simulink model "Model_OLD"  (R2024b)
settings: Solver=VariableStepAuto  StartTime=0.0  StopTime=20  MaxStep=0.001  RelTol=1e-4
values from neighbouring files (symbols this model uses):
  A = 1.1    [RT14e_Parameters.m]    (also in RT15e_Parameters.m = 1.088; RT15evo_Parameters.m = 1.088; SIM_setup.m = 1.12)
  Aero_balance = 55    [RT14e_Parameters.m]    (also in RT15e_Parameters.m; RT15evo_Parameters.m; SIM_setup.m = 0.55)
  air_density = 1.29    [SIM_setup.m]
  Br_coef_of_friction_F = 0.33    [RT14e_Parameters.m]    (also in RT15e_Parameters.m; RT15evo_Parameters.m; SIM_setup.m = 0.25)
  Br_coef_of_friction_R = 0.33    [RT14e_Parameters.m]    (also in RT15e_Parameters.m; RT15evo_Parameters.m; SIM_setup.m = 0.25)
  Br_pistons_area_F = 3617.26/1e6    (= 0.00361726)    [RT14e_Parameters.m]    (also in RT15e_Parameters.m; RT15evo_Parameters.m; SIM_setup.m)
  Br_pistons_area_R = 2026.83/1e6    (= 0.00202683)    [RT14e_Parameters.m]    (also in RT15e_Parameters.m; RT15evo_Parameters.m; SIM_setup.m)
  Cd = 1.387    [SIM_setup.m]
  Cl = 3.299    [SIM_setup.m]
  CoG_z = 0.35    [RT14e_Parameters.m]    (also in RT15e_Parameters.m = 0.28495; RT15evo_Parameters.m = 0.28495; SIM_setup.m = 0.328)
  Default_Fz_F = g*(Mass*(Lr/Wheelbase))    [RT14e_Parameters.m]    (also in RT15e_Parameters.m; RT15evo_Parameters.m; SIM_setup.m = 608.22)
  Default_Fz_R = g*(Mass*(Lf/Wheelbase))    [RT14e_Parameters.m]    (also in RT15e_Parameters.m; RT15evo_Parameters.m; SIM_setup.m = 774.99)
  Effective_br_disk_r_F = 0.0905    [RT14e_Parameters.m]    (also in RT15e_Parameters.m; RT15evo_Parameters.m; SIM_setup.m)
  Effective_br_disk_r_R = 0.0895    [RT14e_Parameters.m]    (also in RT15e_Parameters.m; RT15evo_Parameters.m; SIM_setup.m)
  Front_brake_balance = 0.0    (= 0)    [RT14e_Parameters.m]    (also in RT15e_Parameters.m; RT15evo_Parameters.m)
  Front_brake_pump_area = 153.94    [RT14e_Parameters.m]    (also in RT15e_Parameters.m; RT15evo_Parameters.m)
  Front_desired_brake_p_balance = 0.6    [RT14e_Parameters.m]    (also in RT15e_Parameters.m; RT15evo_Parameters.m)
  Fx = Data_Fx(2:end,3:end)    [RT14e_Parameters.m]    (also in RT15e_Parameters.m; RT15evo_Parameters.m; SIM_setup.m = Data_Fx(2:end,2:end))
  Fy = Data_Fy(2:end,3:end)    [RT14e_Parameters.m]    (also in RT15e_Parameters.m; RT15evo_Parameters.m; SIM_setup.m = Data_Fy(2:end,2:end))
  Fz = Data_Fy(2:end,2)    [RT14e_Parameters.m]    (also in RT15e_Parameters.m; RT15evo_Parameters.m; SIM_setup.m = Data_Fy(2:end,1))
  Half_track = 0.6    [SIM_setup.m]
  Iz_wehicle = 120    [RT14e_Parameters.m]    (also in RT15e_Parameters.m; RT15evo_Parameters.m; SIM_setup.m)
  Iz_wheel = 0.15    [RT14e_Parameters.m]    (also in RT15e_Parameters.m; RT15evo_Parameters.m; SIM_setup.m)
  Lateral_load_transfer_distribution = 0.55    [SIM_setup.m]
  Lf = Wheelbase - CoG_x    (= 0.77)    [RT14e_Parameters.m]    (also in RT15e_Parameters.m = 0.7504; RT15evo_Parameters.m = 0.7504; SIM_setup.m)
  Lock_brake_balance = false    [RT14e_Parameters.m]    (also in RT15e_Parameters.m; RT15evo_Parameters.m)
  Lr = Wheelbase - Lf    (= 0.755)    [RT14e_Parameters.m]    (also in RT15e_Parameters.m = 0.7746; RT15evo_Parameters.m = 0.7746; SIM_setup.m)
  Mass = Vehicle_mass + Driver_mass    (= 290)    [RT14e_Parameters.m]    (also in RT15e_Parameters.m = 265; RT15evo_Parameters.m; SIM_setup.m = 300)
  Max_Torque = 29.1    [SIM_setup.m]
  Motor_maximum_power = 35366    [RT14e_Parameters.m]    (also in RT15e_Parameters.m; RT15evo_Parameters.m)
  RB_torque_setting_1 = -2    [RT14e_Parameters.m]    (also in RT15e_Parameters.m; RT15evo_Parameters.m; SIM_setup.m)
  RB_torque_setting_10 = -20    [RT14e_Parameters.m]    (also in RT15e_Parameters.m; RT15evo_Parameters.m; SIM_setup.m)
  RB_torque_setting_2 = -4    [RT14e_Parameters.m]    (also in RT15e_Parameters.m; RT15evo_Parameters.m; SIM_setup.m)
  RB_torque_setting_3 = -6    [RT14e_Parameters.m]    (also in RT15e_Parameters.m; RT15evo_Parameters.m; SIM_setup.m)
  RB_torque_setting_4 = -8    [RT14e_Parameters.m]    (also in RT15e_Parameters.m; RT15evo_Parameters.m; SIM_setup.m)
  RB_torque_setting_5 = -10    [RT14e_Parameters.m]    (also in RT15e_Parameters.m; RT15evo_Parameters.m; SIM_setup.m)
  RB_torque_setting_6 = -12    [RT14e_Parameters.m]    (also in RT15e_Parameters.m; RT15evo_Parameters.m; SIM_setup.m)
  RB_torque_setting_7 = -14    [RT14e_Parameters.m]    (also in RT15e_Parameters.m; RT15evo_Parameters.m; SIM_setup.m)
  RB_torque_setting_8 = -16    [RT14e_Parameters.m]    (also in RT15e_Parameters.m; RT15evo_Parameters.m; SIM_setup.m)
  RB_torque_setting_9 = -18    [RT14e_Parameters.m]    (also in RT15e_Parameters.m; RT15evo_Parameters.m; SIM_setup.m)
  Rear_brake_pump_area = 198.56    [RT14e_Parameters.m]    (also in RT15e_Parameters.m; RT15evo_Parameters.m)
  SA = Data_Fy(1,3:end)    [RT14e_Parameters.m]    (also in RT15e_Parameters.m; RT15evo_Parameters.m; SIM_setup.m = Data_Fy(1,2:end))
  SR = Data_Fx(1,3:end)    [RT14e_Parameters.m]    (also in RT15e_Parameters.m; RT15evo_Parameters.m; SIM_setup.m = Data_Fx(1,2:end))
  start_time = 182    [SIM_setup.m]
  start_velocity = Xsens_MTI_670_vel.Value(find(Xsens_MTI_670_vel.Time > start_time, 1)) * 1000 / 3600    [SIM_setup.m]
  Steering_angle_table = [0 9.9 19.9 30.14 40.57 51.05 61.29 70.87 79.38 91.9]    [SIM_setup.m]
  Steering_ratio_table = [3.25 3.24 3.23 3.20 3.16 3.10 3.04 2.97 2.90 2.77]    [SIM_setup.m]
  Tire_radius = 0.203    [RT14e_Parameters.m]    (also in RT15e_Parameters.m; RT15evo_Parameters.m; SIM_setup.m)
  Torque_limit_2 = Motor_maximum_torque*0.2    (= 5.82)    [RT14e_Parameters.m]    (also in RT15e_Parameters.m; RT15evo_Parameters.m; SIM_setup.m)
  Torque_limit_3 = Motor_maximum_torque*0.3    (= 8.73)    [RT14e_Parameters.m]    (also in RT15e_Parameters.m; RT15evo_Parameters.m; SIM_setup.m)
  Torque_limit_4 = Motor_maximum_torque*0.4    (= 11.64)    [RT14e_Parameters.m]    (also in RT15e_Parameters.m; RT15evo_Parameters.m; SIM_setup.m)
  Torque_limit_5 = Motor_maximum_torque*0.5    (= 14.55)    [RT14e_Parameters.m]    (also in RT15e_Parameters.m; RT15evo_Parameters.m; SIM_setup.m)
  Torque_limit_6 = Motor_maximum_torque*0.6    (= 17.46)    [RT14e_Parameters.m]    (also in RT15e_Parameters.m; RT15evo_Parameters.m; SIM_setup.m)
  Torque_limit_7 = Motor_maximum_torque*0.7    (= 20.37)    [RT14e_Parameters.m]    (also in RT15e_Parameters.m; RT15evo_Parameters.m; SIM_setup.m)
  Torque_limit_8 = Motor_maximum_torque*0.8    (= 23.28)    [RT14e_Parameters.m]    (also in RT15e_Parameters.m; RT15evo_Parameters.m; SIM_setup.m)
  Torque_limit_9 = 29.1    [RT14e_Parameters.m]    (also in RT15e_Parameters.m; RT15evo_Parameters.m; SIM_setup.m)
  Torque_limit_max = Motor_maximum_torque    (= 29.1)    [RT14e_Parameters.m]    (also in RT15e_Parameters.m; RT15evo_Parameters.m; SIM_setup.m)
  Torque_limit_min = Motor_maximum_torque*0.1    (= 2.91)    [RT14e_Parameters.m]    (also in RT15e_Parameters.m; RT15evo_Parameters.m; SIM_setup.m)
  Transmission_gear_ratio = 12.9    [SIM_setup.m]
  TV_RB_understeer_gradient_1 = -0.5    [RT14e_Parameters.m]    (also in RT15e_Parameters.m; RT15evo_Parameters.m; SIM_setup.m)
  TV_RB_understeer_gradient_10 = 0.005    [RT14e_Parameters.m]    (also in RT15e_Parameters.m; RT15evo_Parameters.m; SIM_setup.m)
  TV_RB_understeer_gradient_2 = -0.1    [RT14e_Parameters.m]    (also in RT15e_Parameters.m; RT15evo_Parameters.m; SIM_setup.m)
  TV_RB_understeer_gradient_3 = 0.08    [RT14e_Parameters.m]    (also in RT15e_Parameters.m; RT15evo_Parameters.m; SIM_setup.m)
  TV_RB_understeer_gradient_4 = 0.06    [RT14e_Parameters.m]    (also in RT15e_Parameters.m; RT15evo_Parameters.m; SIM_setup.m)
  TV_RB_understeer_gradient_5 = 0.05    [RT14e_Parameters.m]    (also in RT15e_Parameters.m; RT15evo_Parameters.m; SIM_setup.m)
  TV_RB_understeer_gradient_6 = 0.04    [RT14e_Parameters.m]    (also in RT15e_Parameters.m; RT15evo_Parameters.m; SIM_setup.m)
  TV_RB_understeer_gradient_7 = 0.03    [RT14e_Parameters.m]    (also in RT15e_Parameters.m; RT15evo_Parameters.m; SIM_setup.m)
  TV_RB_understeer_gradient_8 = 0.02    [RT14e_Parameters.m]    (also in RT15e_Parameters.m; RT15evo_Parameters.m; SIM_setup.m)
  TV_RB_understeer_gradient_9 = 0.01    [RT14e_Parameters.m]    (also in RT15e_Parameters.m; RT15evo_Parameters.m; SIM_setup.m)
  TV_understeer_gradient_1 = -0.5    [RT14e_Parameters.m]    (also in RT15e_Parameters.m; RT15evo_Parameters.m; SIM_setup.m)
  TV_understeer_gradient_10 = 0.002    [RT14e_Parameters.m]    (also in RT15e_Parameters.m; RT15evo_Parameters.m; SIM_setup.m)
  TV_understeer_gradient_2 = -0.1    [RT14e_Parameters.m]    (also in RT15e_Parameters.m; RT15evo_Parameters.m; SIM_setup.m)
  TV_understeer_gradient_3 = 0.06    [RT14e_Parameters.m]    (also in RT15e_Parameters.m; RT15evo_Parameters.m; SIM_setup.m)
  TV_understeer_gradient_4 = 0.05    [RT14e_Parameters.m]    (also in RT15e_Parameters.m; RT15evo_Parameters.m; SIM_setup.m)
  TV_understeer_gradient_5 = 0.04    [RT14e_Parameters.m]    (also in RT15e_Parameters.m; RT15evo_Parameters.m; SIM_setup.m)
  TV_understeer_gradient_6 = 0.03    [RT14e_Parameters.m]    (also in RT15e_Parameters.m; RT15evo_Parameters.m; SIM_setup.m)
  TV_understeer_gradient_7 = 0.02    [RT14e_Parameters.m]    (also in RT15e_Parameters.m; RT15evo_Parameters.m; SIM_setup.m)
  TV_understeer_gradient_8 = 0.01    [RT14e_Parameters.m]    (also in RT15e_Parameters.m; RT15evo_Parameters.m; SIM_setup.m)
  TV_understeer_gradient_9 = 0.005    [RT14e_Parameters.m]    (also in RT15e_Parameters.m; RT15evo_Parameters.m; SIM_setup.m)
  Wheel_base = 1.525    [SIM_setup.m]
  Wheel_rolling_resistance = 0.055    [RT14e_Parameters.m]    (also in RT15e_Parameters.m; RT15evo_Parameters.m; SIM_setup.m)
undefined symbols (not defined in the file or in its folder): Actual_Torque_Value_RL, Actual_Torque_Value_RR, aero_balance, APPS, Brake_Pressure_Front, Brake_Pressure_Rear, lateral_load_transfer_distribution, Steering_position, tire_radius, wheel_base, Wheel_Speed_RL, Wheel_Speed_RR, Xsens_MTI_670_accX, Xsens_MTI_670_accY, Xsens_MTI_670_gyrZ, Xsens_MTI_670_vel, Xsens_Yaw_Rate__deg_s_
libraries: simulink x25, slpidlib x9, simulink_extras x7, dspstat3 x4, slrealtimeloglib x2
(part 2 of 5)

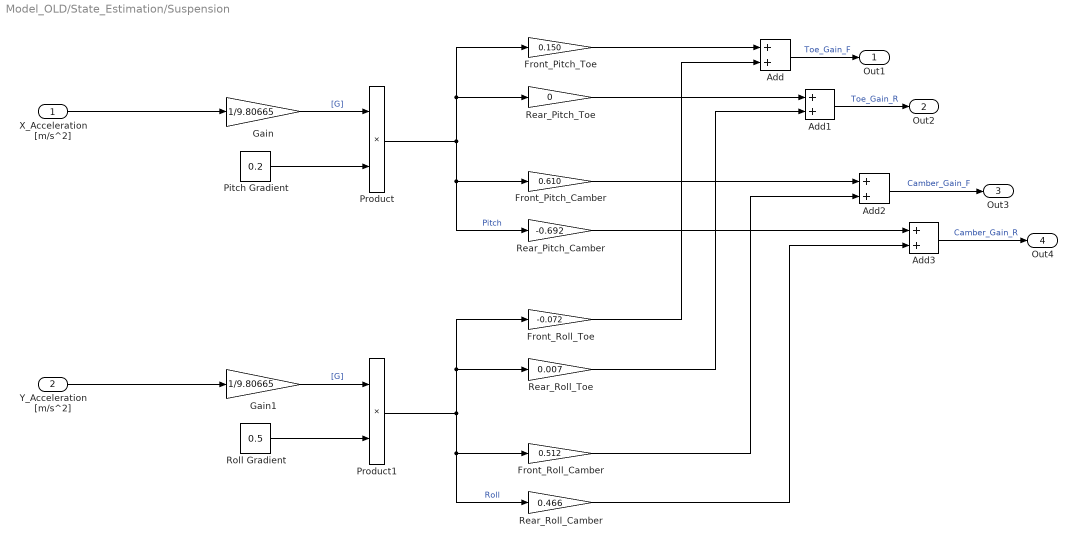
== system Model_OLD/State_Estimation/Suspension ==
  X_Acceleration [m/s^2] : Inport
  Y_Acceleration [m/s^2] : Inport  Port=2
  Add{,1..3} (4 alike) : Sum
  Front_Pitch_Camber : Gain  Gain=0.610
  Front_Pitch_Toe : Gain  Gain=0.150
  Front_Roll_Camber : Gain  Gain=0.512
  Front_Roll_Toe : Gain  Gain=-0.072
  Gain : Gain  Gain=1/9.80665
  Gain1 : Gain  Gain=1/9.80665
  Pitch Gradient : Constant  Value=0.2
  Product : Product
  Product1 : Product
  Rear_Pitch_Camber : Gain  Gain=-0.692
  Rear_Pitch_Toe : Gain  Gain=0
  Rear_Roll_Camber : Gain  Gain=0.466
  Rear_Roll_Toe : Gain  Gain=0.007
  Roll Gradient : Constant  Value=0.5
  Out1 : Outport
  Out2 : Outport  Port=2
  Out3 : Outport  Port=3
  Out4 : Outport  Port=4
  wires:
  Add3/1 -> Out4/1  "Camber_Gain_R"
  Add2/1 -> Out3/1  "Camber_Gain_F"
  Add1/1 -> Out2/1  "Toe_Gain_R"
  Add/1 -> Out1/1  "Toe_Gain_F"
  Rear_Roll_Camber/1 -> Add3/2
  Front_Roll_Camber/1 -> Add2/2
  Rear_Roll_Toe/1 -> Add1/2
  Front_Roll_Toe/1 -> Add/2
  Rear_Pitch_Toe/1 -> Add1/1
  Front_Pitch_Toe/1 -> Add/1
  Rear_Pitch_Camber/1 -> Add3/1
  Front_Pitch_Camber/1 -> Add2/1
  Product/1 -> Rear_Pitch_Toe/1, Front_Pitch_Toe/1, Front_Pitch_Camber/1, Rear_Pitch_Camber/1  "Pitch"
  Product1/1 -> Rear_Roll_Toe/1, Front_Roll_Toe/1, Rear_Roll_Camber/1, Front_Roll_Camber/1  "Roll"
  Gain1/1 -> Product1/1  "[G]"
  Roll Gradient/1 -> Product1/2
  Pitch Gradient/1 -> Product/2
  Y_Acceleration [m/s^2]/1 -> Gain1/1
  Gain/1 -> Product/1  "[G]"
  X_Acceleration [m/s^2]/1 -> Gain/1

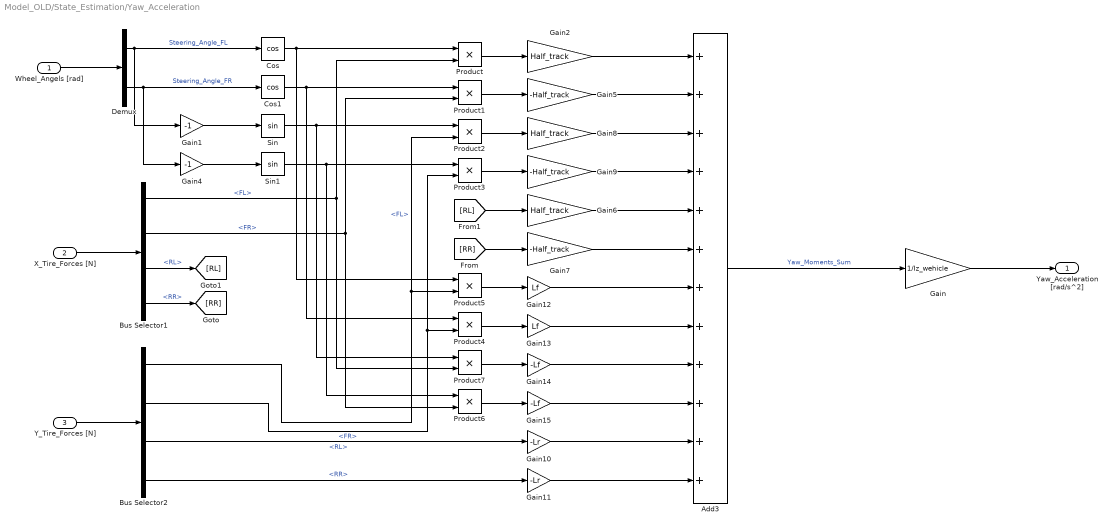
== system Model_OLD/State_Estimation/Yaw_Acceleration ==
  Wheel_Angels [rad] : Inport
  X_Tire_Forces [N] : Inport  Port=2
  Y_Tire_Forces [N] : Inport  Port=3
  Add3 : Sum  Inputs=++++++++++++
  Bus Selector1 : BusSelector  OutputSignals=FL,FR,RL,RR
  Bus Selector2 : BusSelector  OutputSignals=FL,FR,RL,RR
  Cos : Trigonometry  Operator=cos
  Cos1 : Trigonometry  Operator=cos
  Demux : Demux  Outputs=2
  Gain : Gain  Gain=1/Iz_wehicle
  Gain1 : Gain  Gain=-1
  Gain10 : Gain  Gain=-Lr
  Gain11 : Gain  Gain=-Lr
  Gain12 : Gain  Gain=Lf
  Gain13 : Gain  Gain=Lf
  Gain14 : Gain  Gain=-Lf
  Gain15 : Gain  Gain=-Lf
  Gain2 : Gain  Gain=Half_track
  Gain4 : Gain  Gain=-1
  Gain5 : Gain  Gain=-Half_track
  Gain6 : Gain  Gain=Half_track
  Gain7 : Gain  Gain=-Half_track
  Gain8 : Gain  Gain=Half_track
  Gain9 : Gain  Gain=-Half_track
  Product{,1..7} (8 alike) : Product
  Sin : Trigonometry
  Sin1 : Trigonometry
  Yaw_Acceleration [rad/s^2] : Outport
  wires:
  Add3/1 -> Gain/1  "Yaw_Moments_Sum"
  Gain/1 -> Yaw_Acceleration [rad/s^2]/1
  Gain4/1 -> Sin1/1
  Wheel_Angels [rad]/1 -> Demux/1
  Gain1/1 -> Sin/1
  Demux/1 -> Gain1/1, Cos/1  "Steering_Angle_FL"
  Demux/2 -> Cos1/1, Gain4/1  "Steering_Angle_FR"
  Y_Tire_Forces [N]/1 -> Bus Selector2/1
  Cos/1 -> Product/1, Product5/1
  Cos1/1 -> Product1/1, Product4/1
  Product/1 -> Gain2/1
  Product1/1 -> Gain5/1
  Sin/1 -> Product2/1, Product7/1
  Product2/1 -> Gain8/1
  Sin1/1 -> Product3/1, Product6/1
  Product5/1 -> Gain12/1
  Product4/1 -> Gain13/1
  Product6/1 -> Gain15/1
  Product7/1 -> Gain14/1
  X_Tire_Forces [N]/1 -> Bus Selector1/1
  Bus Selector1/2 -> Product6/2, Product1/2  "<FR>"
  Bus Selector1/1 -> Product/2, Product7/2  "<FL>"
  Bus Selector2/2 -> Product4/2, Product3/2  "<FR>"
  Bus Selector2/1 -> Product5/2, Product2/2  "<FL>"
  Gain2/1 -> Add3/1
  Gain5/1 -> Add3/2
  Gain6/1 -> Add3/5
  Gain7/1 -> Add3/6
  Gain8/1 -> Add3/3
  Gain9/1 -> Add3/4
  Product3/1 -> Gain9/1
  Bus Selector2/3 -> Gain10/1  "<RL>"
  Gain10/1 -> Add3/11
  Gain11/1 -> Add3/12
  Bus Selector2/4 -> Gain11/1  "<RR>"
  Gain12/1 -> Add3/7
  Gain13/1 -> Add3/8
  Gain14/1 -> Add3/9
  Gain15/1 -> Add3/10
  [RR] -> Gain7/1
  Bus Selector1/4 -> [RR]  "<RR>"
  [RL] -> Gain6/1
  Bus Selector1/3 -> [RL]  "<RL>"

== system Model_OLD/Tires /FL ==
  In1 : Inport
  2-D Lookup Table : Lookup_n-D  BreakpointsForDimension1=Fz  BreakpointsForDimension2=SA  Table=Fy  InternalRulePriority=Speed  RndMeth=Simplest
      settings: InputPortMap=u0,u1
  2-D Lookup Table1 : Lookup_n-D  BreakpointsForDimension1=Fz  BreakpointsForDimension2=SR  Table=Fx  InternalRulePriority=Speed  RndMeth=Simplest
      settings: InputPortMap=u0,u1
  Bus Selector : BusSelector  OutputSignals=Slip_Ratio.Slip_Ratio_FL,Fz.Fz_FL,Slip_Angle [deg].Slip_Angle_FL
  Fx_FL : Outport
  Fy_FL : Outport  Port=2
  wires:
  2-D Lookup Table/1 -> Fy_FL/1
  2-D Lookup Table1/1 -> Fx_FL/1
  Bus Selector/1 -> 2-D Lookup Table1/2  "<Slip_Ratio_FL>"
  In1/1 -> Bus Selector/1
  Bus Selector/3 -> 2-D Lookup Table/2  "<Slip_Angle_FL>"
  Bus Selector/2 -> 2-D Lookup Table/1, 2-D Lookup Table1/1  "<Fz_FL>"

== system Model_OLD/Tires /FR ==
  In1 : Inport
  2-D Lookup Table : Lookup_n-D  BreakpointsForDimension1=Fz  BreakpointsForDimension2=SA  Table=Fy  InternalRulePriority=Speed  RndMeth=Simplest
      settings: InputPortMap=u0,u1
  2-D Lookup Table1 : Lookup_n-D  BreakpointsForDimension1=Fz  BreakpointsForDimension2=SR  Table=Fx  InternalRulePriority=Speed  RndMeth=Simplest
      settings: InputPortMap=u0,u1
  Bus Selector : BusSelector  OutputSignals=Slip_Ratio.Slip_Ratio_FR,Fz.Fz_FR,Slip_Angle [deg].Slip_Angle_FR
  Fx_FR : Outport
  Fy_FR : Outport  Port=2
  wires:
  2-D Lookup Table1/1 -> Fx_FR/1
  2-D Lookup Table/1 -> Fy_FR/1
  In1/1 -> Bus Selector/1
  Bus Selector/1 -> 2-D Lookup Table1/2  "<Slip_Ratio_FR>"
  Bus Selector/3 -> 2-D Lookup Table/2  "<Slip_Angle_FR>"
  Bus Selector/2 -> 2-D Lookup Table/1, 2-D Lookup Table1/1  "<Fz_FR>"

== system Model_OLD/Tires /RL ==
  In1 : Inport
  2-D Lookup Table : Lookup_n-D  BreakpointsForDimension1=Fz  BreakpointsForDimension2=SA  Table=Fy  InternalRulePriority=Speed  RndMeth=Simplest
      settings: InputPortMap=u0,u1
  2-D Lookup Table1 : Lookup_n-D  BreakpointsForDimension1=Fz  BreakpointsForDimension2=SR  Table=Fx  InternalRulePriority=Speed  RndMeth=Simplest
      settings: InputPortMap=u0,u1
  Bus Selector : BusSelector  OutputSignals=Slip_Ratio.Slip_Ratio_RL,Fz.Fz_RL,Slip_Angle [deg].Slip_Angle_RL
  Fx_RL : Outport
  Fy_RL : Outport  Port=2
  wires:
  2-D Lookup Table/1 -> Fy_RL/1
  In1/1 -> Bus Selector/1
  Bus Selector/1 -> 2-D Lookup Table1/2  "<Slip_Ratio_RL>"
  Bus Selector/3 -> 2-D Lookup Table/2  "<Slip_Angle_RL>"
  Bus Selector/2 -> 2-D Lookup Table1/1, 2-D Lookup Table/1  "<Fz_RL>"
  2-D Lookup Table1/1 -> Fx_RL/1

== system Model_OLD/Tires /RR ==
  In1 : Inport
  2-D Lookup Table : Lookup_n-D  BreakpointsForDimension1=Fz  BreakpointsForDimension2=SA  Table=Fy  InternalRulePriority=Speed  RndMeth=Simplest
      settings: InputPortMap=u0,u1
  2-D Lookup Table1 : Lookup_n-D  BreakpointsForDimension1=Fz  BreakpointsForDimension2=SR  Table=Fx  InternalRulePriority=Speed  RndMeth=Simplest
      settings: InputPortMap=u0,u1
  Bus Selector : BusSelector  OutputSignals=Slip_Ratio.Slip_Ratio_RR,Fz.Fz_RR,Slip_Angle [deg].Slip_Angle_RR
  Fx_RR : Outport
  Fy_RR : Outport  Port=2
  wires:
  In1/1 -> Bus Selector/1
  2-D Lookup Table/1 -> Fy_RR/1
  Bus Selector/1 -> 2-D Lookup Table1/2  "<Slip_Ratio_RR>"
  Bus Selector/3 -> 2-D Lookup Table/2  "<Slip_Angle_RR>"
  Bus Selector/2 -> 2-D Lookup Table/1, 2-D Lookup Table1/1  "<Fz_RR>"
  2-D Lookup Table1/1 -> Fx_RR/1

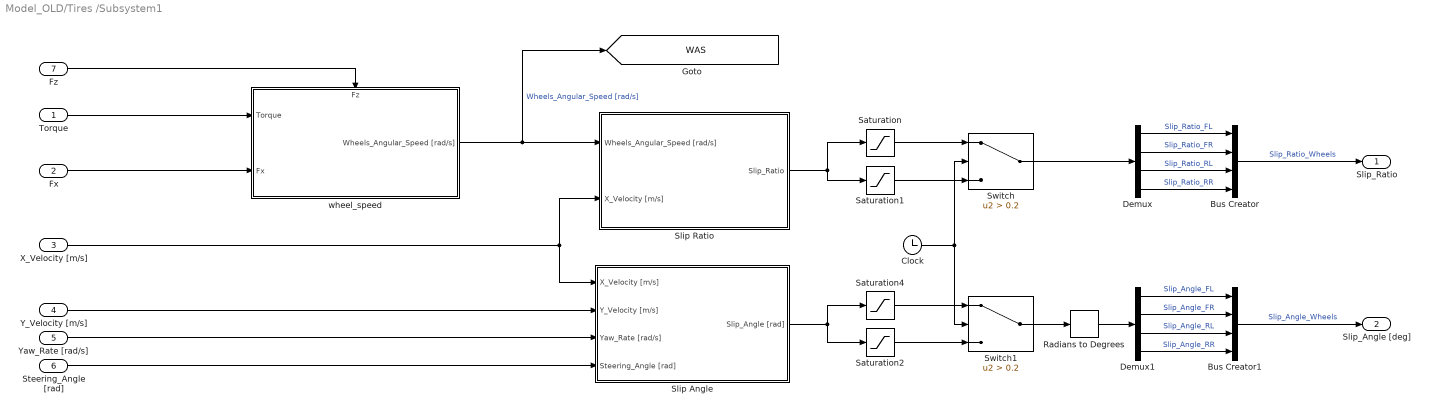
== system Model_OLD/Tires /Subsystem1 ==
  Torque : Inport
  Fx : Inport  Port=2
  X_Velocity [m/s] : Inport  Port=3
  Y_Velocity [m/s] : Inport  Port=4
  Yaw_Rate [rad/s] : Inport  Port=5
  Steering_Angle [rad] : Inport  Port=6
  Fz : Inport  Port=7
  Bus Creator : BusCreator  Inputs=4
  Bus Creator1 : BusCreator  Inputs=4
  Clock : Clock
  Demux : Demux
  Demux1 : Demux
  Radians to Degrees : simulink_extras/Transformations/Radians to Degrees
  Saturation : Saturate  UpperLimit=0.2  LowerLimit=-0.2
  Saturation1 : Saturate  UpperLimit=0.05  LowerLimit=-0.05
  Saturation2 : Saturate  UpperLimit=0.01  LowerLimit=-0.01
  Saturation4 : Saturate  UpperLimit=0.35  LowerLimit=-0.35
  Slip Angle : Subsystem
  Slip Ratio : Subsystem
  Switch : Switch  Criteria=u2 > Threshold  Threshold=0.2  SaturateOnIntegerOverflow=off  InputSameDT=off
  Switch1 : Switch  Criteria=u2 > Threshold  Threshold=0.2  SaturateOnIntegerOverflow=off  InputSameDT=off
  wheel_speed : Subsystem
      settings: PortSchema="{\"entries\":[{\"content\":{\"sides\":[{\"content\":{\"connectorIds\":[\"In1\",\"In2\"]},\"type\":\"ConnectorPlacement.EquallySpacedRectSide\",\"uuid\":\"15092166-14ce-458f-8814-c8c529b404ff\"},{\"content\":{\"connectorIds\":[\"Out1\"],\"side\":\"RIGHT\"},\"type\":\"ConnectorPlacement.EquallySpacedRectSide\",\"uuid\":\"66225d7f-0835-4a54-ba48-dd0fc21c3b18\"},{\"content\":{\"connectorIds\":[\"In3\"],\"side\":\"TOP\"},\"type\":\"ConnectorPlacement.EquallySpacedRectSide\",\"uuid\":\"e640b56a-2f04-4291-8d41-f01328ba15b5\"}]},\"type\":\"ConnectorPlacement.EquallySpacedConnector\",\"uuid\":\"87946f02-b44c-4e08-9031-15e47f027ea8\"}],\"packageUris\":[\"http://schema.mathworks.com/mf0/Connector/R2020b\"],\"version\":\"1.0\"}"
  Slip_Ratio : Outport
  Slip_Angle [deg] : Outport  Port=2
  tag scope: WAS=global
  wires:
  wheel_speed/1(Wheels_Angular_Speed [rad/s]) -> [WAS], Slip Ratio/1(Wheels_Angular_Speed [rad/s])  "Wheels_Angular_Speed [rad/s]"
  X_Velocity [m/s]/1 -> Slip Ratio/2(X_Velocity [m/s]), Slip Angle/1(X_Velocity [m/s])
  Slip Ratio/1(Slip_Ratio) -> Saturation/1, Saturation1/1
  Torque/1 -> wheel_speed/1(Torque)
  Y_Velocity [m/s]/1 -> Slip Angle/2(Y_Velocity [m/s])
  Slip Angle/1(Slip_Angle [rad]) -> Saturation2/1, Saturation4/1
  Steering_Angle [rad]/1 -> Slip Angle/4(Steering_Angle [rad])
  Fx/1 -> wheel_speed/2(Fx)
  Yaw_Rate [rad/s]/1 -> Slip Angle/3(Yaw_Rate [rad/s])
  Demux/1 -> Bus Creator/1  "Slip_Ratio_FL"
  Demux/2 -> Bus Creator/2  "Slip_Ratio_FR"
  Demux/3 -> Bus Creator/3  "Slip_Ratio_RL"
  Demux/4 -> Bus Creator/4  "Slip_Ratio_RR"
  Bus Creator/1 -> Slip_Ratio/1  "Slip_Ratio_Wheels"
  Demux1/4 -> Bus Creator1/4  "Slip_Angle_RR"
  Demux1/3 -> Bus Creator1/3  "Slip_Angle_RL"
  Demux1/2 -> Bus Creator1/2  "Slip_Angle_FR"
  Demux1/1 -> Bus Creator1/1  "Slip_Angle_FL"
  Radians to Degrees/1 -> Demux1/1
  Bus Creator1/1 -> Slip_Angle [deg]/1  "Slip_Angle_Wheels"
  Saturation/1 -> Switch/1
  Saturation1/1 -> Switch/3
  Saturation4/1 -> Switch1/1
  Saturation2/1 -> Switch1/3
  Fz/1 -> wheel_speed/3(Fz)
  Switch1/1 -> Radians to Degrees/1
  Switch/1 -> Demux/1
  Clock/1 -> Switch/2, Switch1/2

== system Model_OLD/Drivetrain/ABS/ABS_FL ==
  Torque IN : Inport
  Slip_Ratio : Inport  Port=2
  Constant : Constant  Value=0.1
  Constant1 : Constant  Value=0.1
  Constant2 : Constant  Value=0.2
  Constant3 : Constant  Value=0
  Constant4 : Constant
  Gain : Gain  Gain=-1
  PID Controller : slpidlib/PID Controller  Controller=PI  Form=Ideal  TimeDomain=Continuous-time  UseExternalTs=off  SampleTime=-1  IntegratorMethod=Forward Euler  FilterMethod=Forward Euler  ControllerParametersSource=internal  P=100  I=10  UseKiTs=on  D=1  UseExternalDerivativeSource=off  N=100  UseFilter=on  TunerSelectOption=Transfer Function Based (PID Tuner App)  InitialConditionSource=internal  InitialConditionForIntegrator=0  InitialConditionForFilter=0  DifferentiatorICPrevScaledInput=0  ExternalReset=none  TrackingMode=off  Kt=1  LimitOutput=off  SatLimitsSource=internal  UpperSaturationLimit=inf  LowerSaturationLimit=-inf  LinearizeAsGain=on  AntiWindupMode=none  Kb=1  LimitIntegrator=off  UpperIntegratorSaturationLimit=inf  LowerIntegratorSaturationLimit=-inf  POutMin=[]  POutMax=[]  IOutMin=[]  IOutMax=[]  DOutMin=[]  DOutMax=[]  NOutMin=[]  NOutMax=[]  SumOutMin=[]  SumOutMax=[]  SaturationOutMin=[]  SaturationOutMax=[]  PParamMin=[]  PParamMax=[]  IParamMin=[]  IParamMax=[]  DParamMin=[]  DParamMax=[]  NParamMin=[]  NParamMax=[]  KbParamMin=[]  KbParamMax=[]  KtParamMin=[]  KtParamMax=[]  KbOutMin=[]  KbOutMax=[]  KtOutMin=[]  KtOutMax=[]  IntegratorOutMin=[]  IntegratorOutMax=[]  FilterOutMin=[]  FilterOutMax=[]  SumI1OutMin=[]  SumI1OutMax=[]  SumI2OutMin=[]  SumI2OutMax=[]  SumI3OutMin=[]  SumI3OutMax=[]  SumI4OutMin=[]  SumI4OutMax=[]  SumDOutMin=[]  SumDOutMax=[]  DifferentiatorOutMin=[]  DifferentiatorOutMax=[]  FilterDiffOutCoefMin=[]  FilterDiffOutCoefMax=[]  ReciprocalOutMin=[]  ReciprocalOutMax=[]  SumDenOutMin=[]  SumDenOutMax=[]  SumNumOutMin=[]  SumNumOutMax=[]  DivideOutMin=[]  DivideOutMax=[]  UdiffTsProdOutMin=[]  UdiffTsProdOutMax=[]  NTsProdOutMin=[]  NTsProdOutMax=[]  UintegralTsProdOutMin=[]  UintegralTsProdOutMax=[]  UngainTsProdOutMin=[]  UngainTsProdOutMax=[]  ClampingZeroOutDataTypeStr=Inherit: Inherit via back propagation  ClampingZeroOutMin=[]  ClampingZeroOutMax=[]  FilterDenConstantOutDataTypeStr=Inherit: Inherit via back propagation  FilterDenConstantOutMin=[]  FilterDenConstantOutMax=[]  PCopyOutDataTypeStr=Inherit: Inherit via back propagation  PCopyOutMin=[]  PCopyOutMax=[]  NCopyOutDataTypeStr=Inherit: Inherit via back propagation  NCopyOutMin=[]  NCopyOutMax=[]  IntegratorContinuousStateAttributes=''  IntegratorStateMustResolveToSignalObject=off  IntegratorRTWStateStorageClass=Auto  FilterContinuousStateAttributes=''  FilterStateMustResolveToSignalObject=off  FilterRTWStateStorageClass=Auto  ParallelPVariant=Passthrough  IdealPVariant=InternalParameters  IVariant=InternalParameters  DVariant=Disabled  IntegratorVariant=Continuous  SatVariant=Disabled  AWVariant=Passthrough  PCopyVariant=Disabled  TRVariant=Disabled  FdbkBlocksVariant=Forward  IdealPFdbkVariant=Disabled  SatFdbkVariant=Disabled  DerivativeFilterVariant=Disabled  NVariant=Disabled  NCopyVariant=Disabled_SignalSpec  FilterICVariant=Disabled  IntegratorICVariant=InternalICs  ExternalResetVariant=Disabled  TRSumVariant=Passthrough  SumFdbkVariant=Disabled  SumVariant=Sum_PI  TsampFilterVariant=InternalTs  TsampNgainVariant=Passthrough  TsampIntegralVariant=Disabled_SignalSpec  ExternalSaturationOutDataTypeStr=Inherit: Same as second input  DerivativeSourceVariant=Disabled  PreIntVariant=InternalPreInt
  Product : Product
  Relational Operator : RelationalOperator  Operator=<=  OutDataTypeStr=boolean  RndMeth=Simplest  InputSameDT=off
  Sum1 : Sum  Inputs=|++
  Switch : Switch  Criteria=u2 > Threshold  SaturateOnIntegerOverflow=off  InputSameDT=off
  Switch1 : Switch  Criteria=u2 > Threshold  SaturateOnIntegerOverflow=off  InputSameDT=off
  Switch2 : Switch  Criteria=u2 > Threshold  SaturateOnIntegerOverflow=off  InputSameDT=off
  ABS Torque OUT : Outport
  wires:
  Product/1 -> ABS Torque OUT/1  "Torq OUT"
  Switch/1 -> Sum1/2  "Ref Slip Ratio"
  Constant/1 -> Relational Operator/1
  Sum1/1 -> Switch1/1  "Slip Ratio Delta"
  Switch1/1 -> PID Controller/1
  PID Controller/1 -> Switch2/1
  Constant2/1 -> Switch/3
  Gain/1 -> Relational Operator/2
  Switch2/1 -> Product/2
  Constant4/1 -> Switch2/3
  Torque IN/1 -> Product/1  "Torque IN"
  Constant1/1 -> Switch/2, Switch/1
  Constant3/1 -> Switch1/3
  Relational Operator/1 -> Switch2/2, Switch1/2
  Slip_Ratio/1 -> Gain/1, Sum1/1  "Slip Ratio"

== system Model_OLD/Drivetrain/ABS/ABS_FR ==
  Torque IN : Inport
  Slip_Ratio : Inport  Port=2
  Constant : Constant  Value=0.1
  Constant1 : Constant  Value=0.1
  Constant2 : Constant  Value=0.2
  Constant3 : Constant  Value=0
  Constant4 : Constant
  Gain : Gain  Gain=-1
  PID Controller : slpidlib/PID Controller  Controller=PI  Form=Ideal  TimeDomain=Continuous-time  UseExternalTs=off  SampleTime=-1  IntegratorMethod=Forward Euler  FilterMethod=Forward Euler  ControllerParametersSource=internal  P=100  I=10  UseKiTs=on  D=1  UseExternalDerivativeSource=off  N=100  UseFilter=on  TunerSelectOption=Transfer Function Based (PID Tuner App)  InitialConditionSource=internal  InitialConditionForIntegrator=0  InitialConditionForFilter=0  DifferentiatorICPrevScaledInput=0  ExternalReset=none  TrackingMode=off  Kt=1  LimitOutput=off  SatLimitsSource=internal  UpperSaturationLimit=inf  LowerSaturationLimit=-inf  LinearizeAsGain=on  AntiWindupMode=none  Kb=1  LimitIntegrator=off  UpperIntegratorSaturationLimit=inf  LowerIntegratorSaturationLimit=-inf  POutMin=[]  POutMax=[]  IOutMin=[]  IOutMax=[]  DOutMin=[]  DOutMax=[]  NOutMin=[]  NOutMax=[]  SumOutMin=[]  SumOutMax=[]  SaturationOutMin=[]  SaturationOutMax=[]  PParamMin=[]  PParamMax=[]  IParamMin=[]  IParamMax=[]  DParamMin=[]  DParamMax=[]  NParamMin=[]  NParamMax=[]  KbParamMin=[]  KbParamMax=[]  KtParamMin=[]  KtParamMax=[]  KbOutMin=[]  KbOutMax=[]  KtOutMin=[]  KtOutMax=[]  IntegratorOutMin=[]  IntegratorOutMax=[]  FilterOutMin=[]  FilterOutMax=[]  SumI1OutMin=[]  SumI1OutMax=[]  SumI2OutMin=[]  SumI2OutMax=[]  SumI3OutMin=[]  SumI3OutMax=[]  SumI4OutMin=[]  SumI4OutMax=[]  SumDOutMin=[]  SumDOutMax=[]  DifferentiatorOutMin=[]  DifferentiatorOutMax=[]  FilterDiffOutCoefMin=[]  FilterDiffOutCoefMax=[]  ReciprocalOutMin=[]  ReciprocalOutMax=[]  SumDenOutMin=[]  SumDenOutMax=[]  SumNumOutMin=[]  SumNumOutMax=[]  DivideOutMin=[]  DivideOutMax=[]  UdiffTsProdOutMin=[]  UdiffTsProdOutMax=[]  NTsProdOutMin=[]  NTsProdOutMax=[]  UintegralTsProdOutMin=[]  UintegralTsProdOutMax=[]  UngainTsProdOutMin=[]  UngainTsProdOutMax=[]  ClampingZeroOutDataTypeStr=Inherit: Inherit via back propagation  ClampingZeroOutMin=[]  ClampingZeroOutMax=[]  FilterDenConstantOutDataTypeStr=Inherit: Inherit via back propagation  FilterDenConstantOutMin=[]  FilterDenConstantOutMax=[]  PCopyOutDataTypeStr=Inherit: Inherit via back propagation  PCopyOutMin=[]  PCopyOutMax=[]  NCopyOutDataTypeStr=Inherit: Inherit via back propagation  NCopyOutMin=[]  NCopyOutMax=[]  IntegratorContinuousStateAttributes=''  IntegratorStateMustResolveToSignalObject=off  IntegratorRTWStateStorageClass=Auto  FilterContinuousStateAttributes=''  FilterStateMustResolveToSignalObject=off  FilterRTWStateStorageClass=Auto  ParallelPVariant=Passthrough  IdealPVariant=InternalParameters  IVariant=InternalParameters  DVariant=Disabled  IntegratorVariant=Continuous  SatVariant=Disabled  AWVariant=Passthrough  PCopyVariant=Disabled  TRVariant=Disabled  FdbkBlocksVariant=Forward  IdealPFdbkVariant=Disabled  SatFdbkVariant=Disabled  DerivativeFilterVariant=Disabled  NVariant=Disabled  NCopyVariant=Disabled_SignalSpec  FilterICVariant=Disabled  IntegratorICVariant=InternalICs  ExternalResetVariant=Disabled  TRSumVariant=Passthrough  SumFdbkVariant=Disabled  SumVariant=Sum_PI  TsampFilterVariant=InternalTs  TsampNgainVariant=Passthrough  TsampIntegralVariant=Disabled_SignalSpec  ExternalSaturationOutDataTypeStr=Inherit: Same as second input  DerivativeSourceVariant=Disabled  PreIntVariant=InternalPreInt
  Product : Product
  Relational Operator : RelationalOperator  Operator=<=  OutDataTypeStr=boolean  RndMeth=Simplest  InputSameDT=off
  Sum1 : Sum  Inputs=|++
  Switch : Switch  Criteria=u2 > Threshold  SaturateOnIntegerOverflow=off  InputSameDT=off
  Switch1 : Switch  Criteria=u2 > Threshold  SaturateOnIntegerOverflow=off  InputSameDT=off
  Switch2 : Switch  Criteria=u2 > Threshold  SaturateOnIntegerOverflow=off  InputSameDT=off
  ABS Torque OUT : Outport
  wires:
  Product/1 -> ABS Torque OUT/1  "Torq OUT"
  Switch/1 -> Sum1/2  "Ref Slip Ratio"
  Constant/1 -> Relational Operator/1
  Sum1/1 -> Switch1/1  "Slip Ratio Delta"
  Switch1/1 -> PID Controller/1
  PID Controller/1 -> Switch2/1
  Constant2/1 -> Switch/3
  Gain/1 -> Relational Operator/2
  Switch2/1 -> Product/2
  Constant4/1 -> Switch2/3
  Torque IN/1 -> Product/1  "Torque IN"
  Constant1/1 -> Switch/2, Switch/1
  Constant3/1 -> Switch1/3
  Relational Operator/1 -> Switch2/2, Switch1/2
  Slip_Ratio/1 -> Gain/1, Sum1/1  "Slip Ratio"

== system Model_OLD/Drivetrain/ABS/ABS_RL ==
  Torque IN : Inport
  Slip_Ratio : Inport  Port=2
  Constant : Constant  Value=0.1
  Constant1 : Constant  Value=0.1
  Constant2 : Constant  Value=0.2
  Constant3 : Constant  Value=0
  Constant4 : Constant
  Gain : Gain  Gain=-1
  PID Controller : slpidlib/PID Controller  Controller=PI  Form=Ideal  TimeDomain=Continuous-time  UseExternalTs=off  SampleTime=-1  IntegratorMethod=Forward Euler  FilterMethod=Forward Euler  ControllerParametersSource=internal  P=100  I=10  UseKiTs=on  D=1  UseExternalDerivativeSource=off  N=100  UseFilter=on  TunerSelectOption=Transfer Function Based (PID Tuner App)  InitialConditionSource=internal  InitialConditionForIntegrator=0  InitialConditionForFilter=0  DifferentiatorICPrevScaledInput=0  ExternalReset=none  TrackingMode=off  Kt=1  LimitOutput=off  SatLimitsSource=internal  UpperSaturationLimit=inf  LowerSaturationLimit=-inf  LinearizeAsGain=on  AntiWindupMode=none  Kb=1  LimitIntegrator=off  UpperIntegratorSaturationLimit=inf  LowerIntegratorSaturationLimit=-inf  POutMin=[]  POutMax=[]  IOutMin=[]  IOutMax=[]  DOutMin=[]  DOutMax=[]  NOutMin=[]  NOutMax=[]  SumOutMin=[]  SumOutMax=[]  SaturationOutMin=[]  SaturationOutMax=[]  PParamMin=[]  PParamMax=[]  IParamMin=[]  IParamMax=[]  DParamMin=[]  DParamMax=[]  NParamMin=[]  NParamMax=[]  KbParamMin=[]  KbParamMax=[]  KtParamMin=[]  KtParamMax=[]  KbOutMin=[]  KbOutMax=[]  KtOutMin=[]  KtOutMax=[]  IntegratorOutMin=[]  IntegratorOutMax=[]  FilterOutMin=[]  FilterOutMax=[]  SumI1OutMin=[]  SumI1OutMax=[]  SumI2OutMin=[]  SumI2OutMax=[]  SumI3OutMin=[]  SumI3OutMax=[]  SumI4OutMin=[]  SumI4OutMax=[]  SumDOutMin=[]  SumDOutMax=[]  DifferentiatorOutMin=[]  DifferentiatorOutMax=[]  FilterDiffOutCoefMin=[]  FilterDiffOutCoefMax=[]  ReciprocalOutMin=[]  ReciprocalOutMax=[]  SumDenOutMin=[]  SumDenOutMax=[]  SumNumOutMin=[]  SumNumOutMax=[]  DivideOutMin=[]  DivideOutMax=[]  UdiffTsProdOutMin=[]  UdiffTsProdOutMax=[]  NTsProdOutMin=[]  NTsProdOutMax=[]  UintegralTsProdOutMin=[]  UintegralTsProdOutMax=[]  UngainTsProdOutMin=[]  UngainTsProdOutMax=[]  ClampingZeroOutDataTypeStr=Inherit: Inherit via back propagation  ClampingZeroOutMin=[]  ClampingZeroOutMax=[]  FilterDenConstantOutDataTypeStr=Inherit: Inherit via back propagation  FilterDenConstantOutMin=[]  FilterDenConstantOutMax=[]  PCopyOutDataTypeStr=Inherit: Inherit via back propagation  PCopyOutMin=[]  PCopyOutMax=[]  NCopyOutDataTypeStr=Inherit: Inherit via back propagation  NCopyOutMin=[]  NCopyOutMax=[]  IntegratorContinuousStateAttributes=''  IntegratorStateMustResolveToSignalObject=off  IntegratorRTWStateStorageClass=Auto  FilterContinuousStateAttributes=''  FilterStateMustResolveToSignalObject=off  FilterRTWStateStorageClass=Auto  ParallelPVariant=Passthrough  IdealPVariant=InternalParameters  IVariant=InternalParameters  DVariant=Disabled  IntegratorVariant=Continuous  SatVariant=Disabled  AWVariant=Passthrough  PCopyVariant=Disabled  TRVariant=Disabled  FdbkBlocksVariant=Forward  IdealPFdbkVariant=Disabled  SatFdbkVariant=Disabled  DerivativeFilterVariant=Disabled  NVariant=Disabled  NCopyVariant=Disabled_SignalSpec  FilterICVariant=Disabled  IntegratorICVariant=InternalICs  ExternalResetVariant=Disabled  TRSumVariant=Passthrough  SumFdbkVariant=Disabled  SumVariant=Sum_PI  TsampFilterVariant=InternalTs  TsampNgainVariant=Passthrough  TsampIntegralVariant=Disabled_SignalSpec  ExternalSaturationOutDataTypeStr=Inherit: Same as second input  DerivativeSourceVariant=Disabled  PreIntVariant=InternalPreInt
  Product : Product
  Relational Operator : RelationalOperator  Operator=<=  OutDataTypeStr=boolean  RndMeth=Simplest  InputSameDT=off
  Sum1 : Sum  Inputs=|++
  Switch : Switch  Criteria=u2 > Threshold  SaturateOnIntegerOverflow=off  InputSameDT=off
  Switch1 : Switch  Criteria=u2 > Threshold  SaturateOnIntegerOverflow=off  InputSameDT=off
  Switch2 : Switch  Criteria=u2 > Threshold  SaturateOnIntegerOverflow=off  InputSameDT=off
  ABS Torque OUT : Outport
  wires:
  Product/1 -> ABS Torque OUT/1  "Torq OUT"
  Switch/1 -> Sum1/2  "Ref Slip Ratio"
  Constant/1 -> Relational Operator/1
  Sum1/1 -> Switch1/1  "Slip Ratio Delta"
  Switch1/1 -> PID Controller/1
  PID Controller/1 -> Switch2/1
  Constant2/1 -> Switch/3
  Gain/1 -> Relational Operator/2
  Switch2/1 -> Product/2
  Constant4/1 -> Switch2/3
  Torque IN/1 -> Product/1  "Torque IN"
  Constant1/1 -> Switch/2, Switch/1
  Constant3/1 -> Switch1/3
  Relational Operator/1 -> Switch2/2, Switch1/2
  Slip_Ratio/1 -> Gain/1, Sum1/1  "Slip Ratio"

== system Model_OLD/Drivetrain/ABS/ABS_RR ==
  Torque IN : Inport
  Slip_Ratio : Inport  Port=2
  Constant : Constant  Value=0.1
  Constant1 : Constant  Value=0.1
  Constant2 : Constant  Value=0.2
  Constant3 : Constant  Value=0
  Constant4 : Constant
  Gain : Gain  Gain=-1
  PID Controller : slpidlib/PID Controller  Controller=PI  Form=Ideal  TimeDomain=Continuous-time  UseExternalTs=off  SampleTime=-1  IntegratorMethod=Forward Euler  FilterMethod=Forward Euler  ControllerParametersSource=internal  P=100  I=10  UseKiTs=on  D=1  UseExternalDerivativeSource=off  N=100  UseFilter=on  TunerSelectOption=Transfer Function Based (PID Tuner App)  InitialConditionSource=internal  InitialConditionForIntegrator=0  InitialConditionForFilter=0  DifferentiatorICPrevScaledInput=0  ExternalReset=none  TrackingMode=off  Kt=1  LimitOutput=off  SatLimitsSource=internal  UpperSaturationLimit=inf  LowerSaturationLimit=-inf  LinearizeAsGain=on  AntiWindupMode=none  Kb=1  LimitIntegrator=off  UpperIntegratorSaturationLimit=inf  LowerIntegratorSaturationLimit=-inf  POutMin=[]  POutMax=[]  IOutMin=[]  IOutMax=[]  DOutMin=[]  DOutMax=[]  NOutMin=[]  NOutMax=[]  SumOutMin=[]  SumOutMax=[]  SaturationOutMin=[]  SaturationOutMax=[]  PParamMin=[]  PParamMax=[]  IParamMin=[]  IParamMax=[]  DParamMin=[]  DParamMax=[]  NParamMin=[]  NParamMax=[]  KbParamMin=[]  KbParamMax=[]  KtParamMin=[]  KtParamMax=[]  KbOutMin=[]  KbOutMax=[]  KtOutMin=[]  KtOutMax=[]  IntegratorOutMin=[]  IntegratorOutMax=[]  FilterOutMin=[]  FilterOutMax=[]  SumI1OutMin=[]  SumI1OutMax=[]  SumI2OutMin=[]  SumI2OutMax=[]  SumI3OutMin=[]  SumI3OutMax=[]  SumI4OutMin=[]  SumI4OutMax=[]  SumDOutMin=[]  SumDOutMax=[]  DifferentiatorOutMin=[]  DifferentiatorOutMax=[]  FilterDiffOutCoefMin=[]  FilterDiffOutCoefMax=[]  ReciprocalOutMin=[]  ReciprocalOutMax=[]  SumDenOutMin=[]  SumDenOutMax=[]  SumNumOutMin=[]  SumNumOutMax=[]  DivideOutMin=[]  DivideOutMax=[]  UdiffTsProdOutMin=[]  UdiffTsProdOutMax=[]  NTsProdOutMin=[]  NTsProdOutMax=[]  UintegralTsProdOutMin=[]  UintegralTsProdOutMax=[]  UngainTsProdOutMin=[]  UngainTsProdOutMax=[]  ClampingZeroOutDataTypeStr=Inherit: Inherit via back propagation  ClampingZeroOutMin=[]  ClampingZeroOutMax=[]  FilterDenConstantOutDataTypeStr=Inherit: Inherit via back propagation  FilterDenConstantOutMin=[]  FilterDenConstantOutMax=[]  PCopyOutDataTypeStr=Inherit: Inherit via back propagation  PCopyOutMin=[]  PCopyOutMax=[]  NCopyOutDataTypeStr=Inherit: Inherit via back propagation  NCopyOutMin=[]  NCopyOutMax=[]  IntegratorContinuousStateAttributes=''  IntegratorStateMustResolveToSignalObject=off  IntegratorRTWStateStorageClass=Auto  FilterContinuousStateAttributes=''  FilterStateMustResolveToSignalObject=off  FilterRTWStateStorageClass=Auto  ParallelPVariant=Passthrough  IdealPVariant=InternalParameters  IVariant=InternalParameters  DVariant=Disabled  IntegratorVariant=Continuous  SatVariant=Disabled  AWVariant=Passthrough  PCopyVariant=Disabled  TRVariant=Disabled  FdbkBlocksVariant=Forward  IdealPFdbkVariant=Disabled  SatFdbkVariant=Disabled  DerivativeFilterVariant=Disabled  NVariant=Disabled  NCopyVariant=Disabled_SignalSpec  FilterICVariant=Disabled  IntegratorICVariant=InternalICs  ExternalResetVariant=Disabled  TRSumVariant=Passthrough  SumFdbkVariant=Disabled  SumVariant=Sum_PI  TsampFilterVariant=InternalTs  TsampNgainVariant=Passthrough  TsampIntegralVariant=Disabled_SignalSpec  ExternalSaturationOutDataTypeStr=Inherit: Same as second input  DerivativeSourceVariant=Disabled  PreIntVariant=InternalPreInt
  Product : Product
  Relational Operator : RelationalOperator  Operator=<=  OutDataTypeStr=boolean  RndMeth=Simplest  InputSameDT=off
  Sum1 : Sum  Inputs=|++
  Switch : Switch  Criteria=u2 > Threshold  SaturateOnIntegerOverflow=off  InputSameDT=off
  Switch1 : Switch  Criteria=u2 > Threshold  SaturateOnIntegerOverflow=off  InputSameDT=off
  Switch2 : Switch  Criteria=u2 > Threshold  SaturateOnIntegerOverflow=off  InputSameDT=off
  ABS Torque OUT : Outport
  wires:
  Product/1 -> ABS Torque OUT/1  "Torq OUT"
  Switch/1 -> Sum1/2  "Ref Slip Ratio"
  Constant/1 -> Relational Operator/1
  Sum1/1 -> Switch1/1  "Slip Ratio Delta"
  Switch1/1 -> PID Controller/1
  PID Controller/1 -> Switch2/1
  Constant2/1 -> Switch/3
  Gain/1 -> Relational Operator/2
  Switch2/1 -> Product/2
  Constant4/1 -> Switch2/3
  Torque IN/1 -> Product/1  "Torque IN"
  Constant1/1 -> Switch/2, Switch/1
  Constant3/1 -> Switch1/3
  Relational Operator/1 -> Switch2/2, Switch1/2
  Slip_Ratio/1 -> Gain/1, Sum1/1  "Slip Ratio"

== system Model_OLD/Drivetrain/ABS1/ABS_FL1 ==
  Torque IN : Inport
  Slip_Ratio : Inport  Port=2
  Constant1 : Constant  Value=0.15
  Constant2 : Constant  Value=0.3
  Gain : Gain  Gain=-1
  PID Controller : slpidlib/PID Controller  Controller=PI  Form=Ideal  TimeDomain=Continuous-time  UseExternalTs=off  SampleTime=-1  IntegratorMethod=Forward Euler  FilterMethod=Forward Euler  ControllerParametersSource=internal  P=50  I=2.5  UseKiTs=on  D=1  UseExternalDerivativeSource=off  N=100  UseFilter=on  TunerSelectOption=Transfer Function Based (PID Tuner App)  InitialConditionSource=internal  InitialConditionForIntegrator=0  InitialConditionForFilter=0  DifferentiatorICPrevScaledInput=0  ExternalReset=none  TrackingMode=off  Kt=1  LimitOutput=off  SatLimitsSource=internal  UpperSaturationLimit=inf  LowerSaturationLimit=-inf  LinearizeAsGain=on  AntiWindupMode=none  Kb=1  LimitIntegrator=off  UpperIntegratorSaturationLimit=inf  LowerIntegratorSaturationLimit=-inf  POutMin=[]  POutMax=[]  IOutMin=[]  IOutMax=[]  DOutMin=[]  DOutMax=[]  NOutMin=[]  NOutMax=[]  SumOutMin=[]  SumOutMax=[]  SaturationOutMin=[]  SaturationOutMax=[]  PParamMin=[]  PParamMax=[]  IParamMin=[]  IParamMax=[]  DParamMin=[]  DParamMax=[]  NParamMin=[]  NParamMax=[]  KbParamMin=[]  KbParamMax=[]  KtParamMin=[]  KtParamMax=[]  KbOutMin=[]  KbOutMax=[]  KtOutMin=[]  KtOutMax=[]  IntegratorOutMin=[]  IntegratorOutMax=[]  FilterOutMin=[]  FilterOutMax=[]  SumI1OutMin=[]  SumI1OutMax=[]  SumI2OutMin=[]  SumI2OutMax=[]  SumI3OutMin=[]  SumI3OutMax=[]  SumI4OutMin=[]  SumI4OutMax=[]  SumDOutMin=[]  SumDOutMax=[]  DifferentiatorOutMin=[]  DifferentiatorOutMax=[]  FilterDiffOutCoefMin=[]  FilterDiffOutCoefMax=[]  ReciprocalOutMin=[]  ReciprocalOutMax=[]  SumDenOutMin=[]  SumDenOutMax=[]  SumNumOutMin=[]  SumNumOutMax=[]  DivideOutMin=[]  DivideOutMax=[]  UdiffTsProdOutMin=[]  UdiffTsProdOutMax=[]  NTsProdOutMin=[]  NTsProdOutMax=[]  UintegralTsProdOutMin=[]  UintegralTsProdOutMax=[]  UngainTsProdOutMin=[]  UngainTsProdOutMax=[]  ClampingZeroOutDataTypeStr=Inherit: Inherit via back propagation  ClampingZeroOutMin=[]  ClampingZeroOutMax=[]  FilterDenConstantOutDataTypeStr=Inherit: Inherit via back propagation  FilterDenConstantOutMin=[]  FilterDenConstantOutMax=[]  PCopyOutDataTypeStr=Inherit: Inherit via back propagation  PCopyOutMin=[]  PCopyOutMax=[]  NCopyOutDataTypeStr=Inherit: Inherit via back propagation  NCopyOutMin=[]  NCopyOutMax=[]  IntegratorContinuousStateAttributes=''  IntegratorStateMustResolveToSignalObject=off  IntegratorRTWStateStorageClass=Auto  FilterContinuousStateAttributes=''  FilterStateMustResolveToSignalObject=off  FilterRTWStateStorageClass=Auto  ParallelPVariant=Passthrough  IdealPVariant=InternalParameters  IVariant=InternalParameters  DVariant=Disabled  IntegratorVariant=Continuous  SatVariant=Disabled  AWVariant=Passthrough  PCopyVariant=Disabled  TRVariant=Disabled  FdbkBlocksVariant=Forward  IdealPFdbkVariant=Disabled  SatFdbkVariant=Disabled  DerivativeFilterVariant=Disabled  NVariant=Disabled  NCopyVariant=Disabled_SignalSpec  FilterICVariant=Disabled  IntegratorICVariant=InternalICs  ExternalResetVariant=Disabled  TRSumVariant=Passthrough  SumFdbkVariant=Disabled  SumVariant=Sum_PI  TsampFilterVariant=InternalTs  TsampNgainVariant=Passthrough  TsampIntegralVariant=Disabled_SignalSpec  ExternalSaturationOutDataTypeStr=Inherit: Same as second input  DerivativeSourceVariant=Disabled  PreIntVariant=InternalPreInt
  Product : Product
  Saturation : Saturate  UpperLimit=5  LowerLimit=-5
  Scope : Scope
  Sum1 : Sum  Inputs=|++
  Switch : Switch  Criteria=u2 > Threshold  SaturateOnIntegerOverflow=off  InputSameDT=off
  ABS Torque OUT : Outport
  wires:
  Switch/1 -> Sum1/2  "Ref Slip Ratio"
  Product/1 -> ABS Torque OUT/1  "Torq OUT"
  PID Controller/1 -> Scope/1, Saturation/1
  Slip_Ratio/1 -> Gain/1  "Slip Ratio"
  Constant1/1 -> Switch/2, Switch/1
  Torque IN/1 -> Product/1  "Torque IN"
  Sum1/1 -> PID Controller/1  "Slip Ratio Delta"
  Constant2/1 -> Switch/3
  Saturation/1 -> Product/2
  Gain/1 -> Sum1/1

== system Model_OLD/Drivetrain/ABS1/ABS_FR1 ==
  Torque IN : Inport
  Slip_Ratio : Inport  Port=2
  Constant1 : Constant  Value=0.15
  Constant2 : Constant  Value=0.3
  Gain : Gain  Gain=-1
  PID Controller : slpidlib/PID Controller  Controller=PI  Form=Ideal  TimeDomain=Continuous-time  UseExternalTs=off  SampleTime=-1  IntegratorMethod=Forward Euler  FilterMethod=Forward Euler  ControllerParametersSource=internal  P=50  I=2.5  UseKiTs=on  D=1  UseExternalDerivativeSource=off  N=100  UseFilter=on  TunerSelectOption=Transfer Function Based (PID Tuner App)  InitialConditionSource=internal  InitialConditionForIntegrator=0  InitialConditionForFilter=0  DifferentiatorICPrevScaledInput=0  ExternalReset=none  TrackingMode=off  Kt=1  LimitOutput=off  SatLimitsSource=internal  UpperSaturationLimit=inf  LowerSaturationLimit=-inf  LinearizeAsGain=on  AntiWindupMode=none  Kb=1  LimitIntegrator=off  UpperIntegratorSaturationLimit=inf  LowerIntegratorSaturationLimit=-inf  POutMin=[]  POutMax=[]  IOutMin=[]  IOutMax=[]  DOutMin=[]  DOutMax=[]  NOutMin=[]  NOutMax=[]  SumOutMin=[]  SumOutMax=[]  SaturationOutMin=[]  SaturationOutMax=[]  PParamMin=[]  PParamMax=[]  IParamMin=[]  IParamMax=[]  DParamMin=[]  DParamMax=[]  NParamMin=[]  NParamMax=[]  KbParamMin=[]  KbParamMax=[]  KtParamMin=[]  KtParamMax=[]  KbOutMin=[]  KbOutMax=[]  KtOutMin=[]  KtOutMax=[]  IntegratorOutMin=[]  IntegratorOutMax=[]  FilterOutMin=[]  FilterOutMax=[]  SumI1OutMin=[]  SumI1OutMax=[]  SumI2OutMin=[]  SumI2OutMax=[]  SumI3OutMin=[]  SumI3OutMax=[]  SumI4OutMin=[]  SumI4OutMax=[]  SumDOutMin=[]  SumDOutMax=[]  DifferentiatorOutMin=[]  DifferentiatorOutMax=[]  FilterDiffOutCoefMin=[]  FilterDiffOutCoefMax=[]  ReciprocalOutMin=[]  ReciprocalOutMax=[]  SumDenOutMin=[]  SumDenOutMax=[]  SumNumOutMin=[]  SumNumOutMax=[]  DivideOutMin=[]  DivideOutMax=[]  UdiffTsProdOutMin=[]  UdiffTsProdOutMax=[]  NTsProdOutMin=[]  NTsProdOutMax=[]  UintegralTsProdOutMin=[]  UintegralTsProdOutMax=[]  UngainTsProdOutMin=[]  UngainTsProdOutMax=[]  ClampingZeroOutDataTypeStr=Inherit: Inherit via back propagation  ClampingZeroOutMin=[]  ClampingZeroOutMax=[]  FilterDenConstantOutDataTypeStr=Inherit: Inherit via back propagation  FilterDenConstantOutMin=[]  FilterDenConstantOutMax=[]  PCopyOutDataTypeStr=Inherit: Inherit via back propagation  PCopyOutMin=[]  PCopyOutMax=[]  NCopyOutDataTypeStr=Inherit: Inherit via back propagation  NCopyOutMin=[]  NCopyOutMax=[]  IntegratorContinuousStateAttributes=''  IntegratorStateMustResolveToSignalObject=off  IntegratorRTWStateStorageClass=Auto  FilterContinuousStateAttributes=''  FilterStateMustResolveToSignalObject=off  FilterRTWStateStorageClass=Auto  ParallelPVariant=Passthrough  IdealPVariant=InternalParameters  IVariant=InternalParameters  DVariant=Disabled  IntegratorVariant=Continuous  SatVariant=Disabled  AWVariant=Passthrough  PCopyVariant=Disabled  TRVariant=Disabled  FdbkBlocksVariant=Forward  IdealPFdbkVariant=Disabled  SatFdbkVariant=Disabled  DerivativeFilterVariant=Disabled  NVariant=Disabled  NCopyVariant=Disabled_SignalSpec  FilterICVariant=Disabled  IntegratorICVariant=InternalICs  ExternalResetVariant=Disabled  TRSumVariant=Passthrough  SumFdbkVariant=Disabled  SumVariant=Sum_PI  TsampFilterVariant=InternalTs  TsampNgainVariant=Passthrough  TsampIntegralVariant=Disabled_SignalSpec  ExternalSaturationOutDataTypeStr=Inherit: Same as second input  DerivativeSourceVariant=Disabled  PreIntVariant=InternalPreInt
  Product : Product
  Saturation : Saturate  UpperLimit=5  LowerLimit=-5
  Scope : Scope
  Sum1 : Sum  Inputs=|++
  Switch : Switch  Criteria=u2 > Threshold  SaturateOnIntegerOverflow=off  InputSameDT=off
  ABS Torque OUT : Outport
  wires:
  Constant1/1 -> Switch/2, Switch/1
  Switch/1 -> Sum1/2  "Ref Slip Ratio"
  Constant2/1 -> Switch/3
  Sum1/1 -> PID Controller/1  "Slip Ratio Delta"
  Torque IN/1 -> Product/1  "Torque IN"
  Product/1 -> ABS Torque OUT/1  "Torq OUT"
  Slip_Ratio/1 -> Gain/1  "Slip Ratio"
  PID Controller/1 -> Scope/1, Saturation/1
  Saturation/1 -> Product/2
  Gain/1 -> Sum1/1
